simulink model "chap9_6sim"  (Simulink 8.1)
settings: Solver=ode45  StartTime=0.0  StopTime=10  RelTol=1e-5
settings Model: Creator=hp  LastModifiedBy=liujk  ExtModeTrigMode=oneshot  ExtModeArmWhenConnect=off
settings DataIOCC: LimitDataPoints=off  SignalLoggingName=sigsOut
settings OptimizationCC: BooleanDataType=off  InitFltsAndDblsToZero=on
settings DebuggingCC: SaveWithParameterizedLinksMsg=none  SignalResolutionControl=TryResolveAllWithWarning  SolverPrmCheckMsg=none  MultiTaskDSMMsg=warning  MultiTaskCondExecSysMsg=none  StrictBusMsg=None
settings HardwareCC: TargetUnknown=on
settings RTWCC: IncludeERTFirstTime=on
settings GRTTargetCC: TargetFcnLib=ansi_tfl_tmw.mat

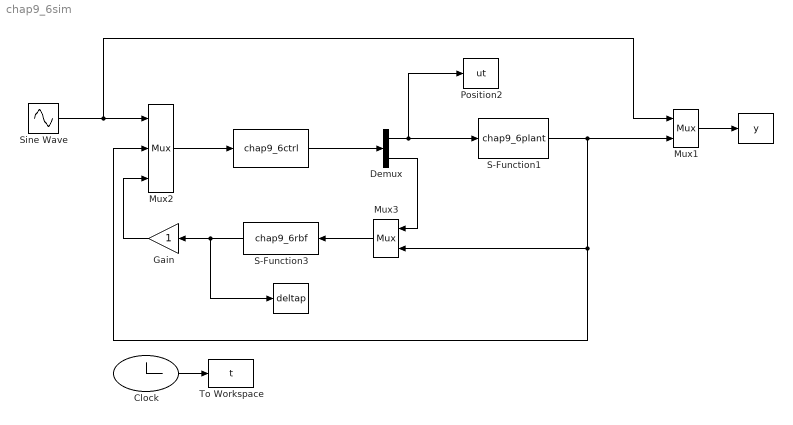
== system chap9_6sim ==
  " " : ToWorkspace  VariableName=deltap  SampleTime=-1
  "  " : ToWorkspace  VariableName=y  SampleTime=-1
  "   " : S-Function  FunctionName=chap9_6ctrl  EnableBusSupport=off
  Clock : Clock
  Demux : Demux  Outputs=2
  Gain : Gain
  Mux1 : Mux  Inputs=2
  Mux2 : Mux  Inputs=3
  Mux3 : Mux  Inputs=2
  Position2 : ToWorkspace  VariableName=ut  SampleTime=-1
  S-Function1 : S-Function  FunctionName=chap9_6plant  EnableBusSupport=off
  S-Function3 : S-Function  FunctionName=chap9_6rbf  EnableBusSupport=off
  Sine Wave : Sin  SampleTime=0
  To Workspace : ToWorkspace  VariableName=t  SampleTime=-1
  wires:
  Mux1/1 -> "  "/1
  Clock/1 -> To Workspace/1
  Sine Wave/1 -> Mux2/1, Mux1/1
  Mux2/1 -> "   "/1
  S-Function3/1 -> " "/1, Gain/1
  Demux/1 -> Position2/1, S-Function1/1
  "   "/1 -> Demux/1
  Mux3/1 -> S-Function3/1
  Demux/2 -> Mux3/1
  S-Function1/1 -> Mux2/2, Mux3/2, Mux1/2
  Gain/1 -> Mux2/3
